simulink model "Validation_Kalman_Filters"  (R2019a)
settings: Solver=ode1  StartTime=0.0  StopTime=100  FixedStep=sampleTime  RelTol=1e-3
values from neighbouring files (symbols this model uses):
  bias = [0; 0; 1]    [Replay_Script.m]    (also in Validations_Script.m = [5; -3; 3]*pi/180)
  filter = d    [Replay_Script.m]    (also in Validations_Script.m = 3)
  Kalman_1 = Kalman_1_theta    [Replay_Script.m]    (also in Validations_Script.m = Setup_Kalman_1(Q, R, sampleTime))
  Kalman_2 = Kalman_2_theta    [Replay_Script.m]    (also in Validations_Script.m = Setup_Kalman_2(Q, R, sampleTime))
  Kalman_OP = Setup_Kalman_OP(Q, R)    [Replay_Script.m]    (also in Validations_Script.m)
  sampleTime = 0.05    [Replay_Script.m]    (also in Validations_Script.m)
undefined symbols (not defined in the file or in its folder): DiscIntNeverNeededParam
libraries: simulink x3
settings Model: Creator=Gaming  LastModifiedBy=Gaming

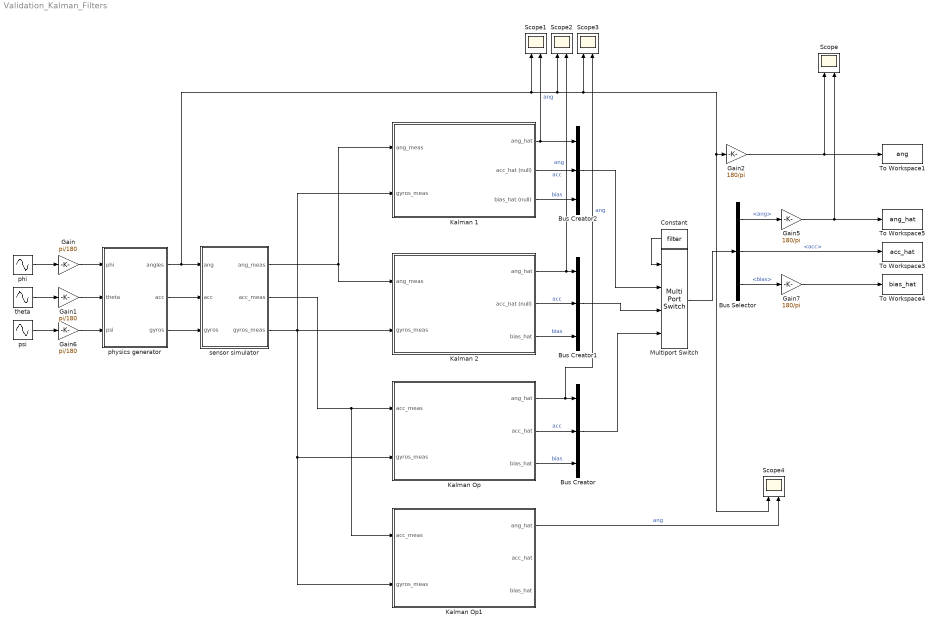
== system Validation_Kalman_Filters ==
  Bus Creator : BusCreator  Inputs=3
  Bus Creator1 : BusCreator  Inputs=3
  Bus Creator2 : BusCreator  Inputs=3
  Bus Selector : BusSelector  OutputSignals=ang,acc,bias
  Constant : Constant  Value=filter
  Gain : Gain  Gain=pi/180
  Gain1 : Gain  Gain=pi/180
  Gain2 : Gain  Gain=180/pi
  Gain5 : Gain  Gain=180/pi
  Gain6 : Gain  Gain=pi/180
  Gain7 : Gain  Gain=180/pi
  Kalman 1 : Subsystem
  Kalman 2 : Subsystem
  Kalman Op : Subsystem
  Kalman Op1 : Subsystem
  Multiport Switch : MultiPortSwitch  AllowDiffInputSizes=on
  Scope{,1..4} (5 alike) : Scope  NumInputPorts=2
  To Workspace1 : ToWorkspace  VariableName=ang  SaveFormat=Structure With Time  SampleTime=-1
  To Workspace3 : ToWorkspace  VariableName=acc_hat  SaveFormat=Structure With Time  SampleTime=-1
  To Workspace4 : ToWorkspace  VariableName=bias_hat  SaveFormat=Structure With Time  SampleTime=-1
  To Workspace5 : ToWorkspace  VariableName=ang_hat  SaveFormat=Structure With Time  SampleTime=-1
  phi : Sin  Amplitude=5  Bias=6  Frequency=2*pi/10  SampleTime=0
  physics generator : Subsystem
  psi : Sin  Amplitude=0  Bias=10  Frequency=2*pi/5  Phase=pi  SampleTime=0
  sensor simulator : Subsystem
  theta : Sin  Amplitude=10  Frequency=2*pi/5  Phase=pi  SampleTime=0
  wires:
  phi/1 -> Gain/1
  theta/1 -> Gain1/1
  Kalman Op/3(bias_hat) -> Bus Creator/3  "bias"
  Kalman Op/1(ang_hat) -> Scope3/2, Bus Creator/1  "ang"
  psi/1 -> Gain6/1
  Gain/1 -> physics generator/1(phi)
  Gain1/1 -> physics generator/2(theta)
  Gain6/1 -> physics generator/3(psi)
  physics generator/1(angles) -> sensor simulator/1(ang), Scope4/1, Gain2/1, Scope3/1, Scope2/1, Scope1/1
  physics generator/2(acc) -> sensor simulator/2(acc)
  physics generator/3(gyros) -> sensor simulator/3(gyros)
  Multiport Switch/1 -> Bus Selector/1
  Gain5/1 -> Scope/2, To Workspace5/1
  Gain7/1 -> To Workspace4/1
  Bus Selector/2 -> To Workspace3/1  "<acc>"
  Kalman Op/2(acc_hat) -> Bus Creator/2  "acc"
  Constant/1 -> Multiport Switch/1
  sensor simulator/2(acc_meas) -> Kalman Op1/1(acc_meas), Kalman Op/1(acc_meas)
  sensor simulator/3(gyros_meas) -> Kalman 2/2(gyros_meas), Kalman 1/2(gyros_meas), Kalman Op/2(gyros_meas), Kalman Op1/2(gyros_meas)
  Bus Selector/1 -> Gain5/1  "<ang>"
  Bus Selector/3 -> Gain7/1  "<bias>"
  Gain2/1 -> To Workspace1/1, Scope/1
  Bus Creator/1 -> Multiport Switch/4
  sensor simulator/1(ang_meas) -> Kalman 2/1(ang_meas), Kalman 1/1(ang_meas)
  Bus Creator1/1 -> Multiport Switch/3
  Bus Creator2/1 -> Multiport Switch/2
  Kalman 1/1(ang_hat) -> Bus Creator2/1, Scope1/2  "ang"
  Kalman 2/1(ang_hat) -> Scope2/2, Bus Creator1/1  "ang"
  Kalman 1/2(acc_hat (null)) -> Bus Creator2/2  "acc"
  Kalman 1/3(bias_hat (null)) -> Bus Creator2/3  "bias"
  Kalman 2/2(acc_hat (null)) -> Bus Creator1/2  "acc"
  Kalman 2/3(bias_hat) -> Bus Creator1/3  "bias"
  Kalman Op1/1(ang_hat) -> Scope4/2  "ang"

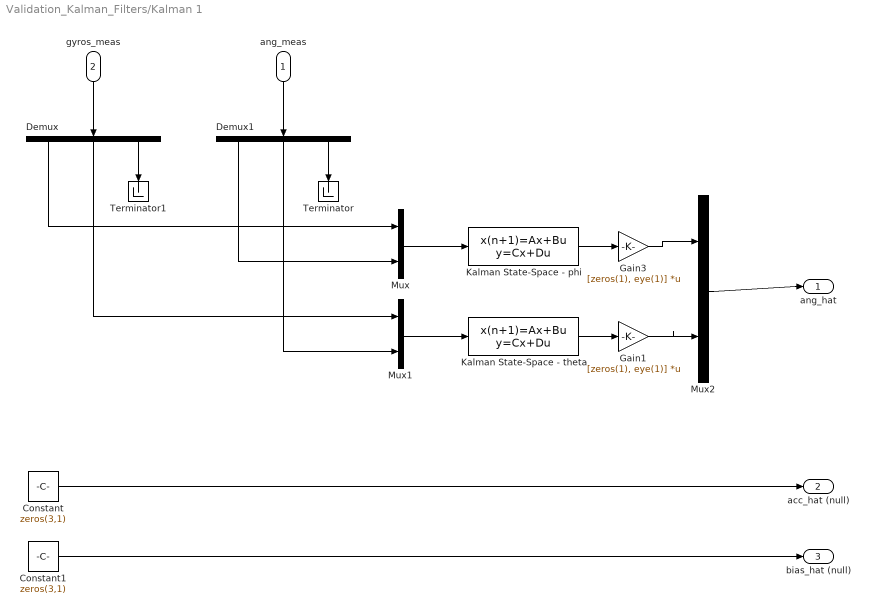
== system Validation_Kalman_Filters/Kalman 1 ==
  ang_meas : Inport
  gyros_meas : Inport  Port=2
  Constant : Constant  Value=zeros(3,1)
  Constant1 : Constant  Value=zeros(3,1)
  Demux : Demux  Outputs=3
  Demux1 : Demux  Outputs=3
  Gain1 : Gain  Gain=[zeros(1), eye(1)]  Multiplication=Matrix(K*u)
  Gain3 : Gain  Gain=[zeros(1), eye(1)]  Multiplication=Matrix(K*u)
  Kalman State-Space - phi : DiscreteStateSpace  A=Kalman_1.sys.A  B=Kalman_1.sys.B  C=Kalman_1.sys.C  D=Kalman_1.sys.D  SampleTime=-1
  Kalman State-Space - theta : DiscreteStateSpace  A=Kalman_1.sys.A  B=Kalman_1.sys.B  C=Kalman_1.sys.C  D=Kalman_1.sys.D  SampleTime=-1
  Mux : Mux  Inputs=2
  Mux1 : Mux  Inputs=2
  Mux2 : Mux  Inputs=2
  Terminator : Terminator
  Terminator1 : Terminator
  ang_hat : Outport  VectorParamsAs1DForOutWhenUnconnected=on
  acc_hat (null) : Outport  Port=2  VectorParamsAs1DForOutWhenUnconnected=on
  bias_hat (null) : Outport  Port=3  VectorParamsAs1DForOutWhenUnconnected=on
  wires:
  Kalman State-Space - phi/1 -> Gain3/1
  Mux/1 -> Kalman State-Space - phi/1
  Constant/1 -> acc_hat (null)/1
  Constant1/1 -> bias_hat (null)/1
  gyros_meas/1 -> Demux/1
  Kalman State-Space - theta/1 -> Gain1/1
  Mux1/1 -> Kalman State-Space - theta/1
  Mux2/1 -> ang_hat/1
  Gain3/1 -> Mux2/1
  Gain1/1 -> Mux2/2
  ang_meas/1 -> Demux1/1
  Demux1/3 -> Terminator/1
  Demux1/2 -> Mux1/2
  Demux1/1 -> Mux/2
  Demux/3 -> Terminator1/1
  Demux/1 -> Mux/1
  Demux/2 -> Mux1/1

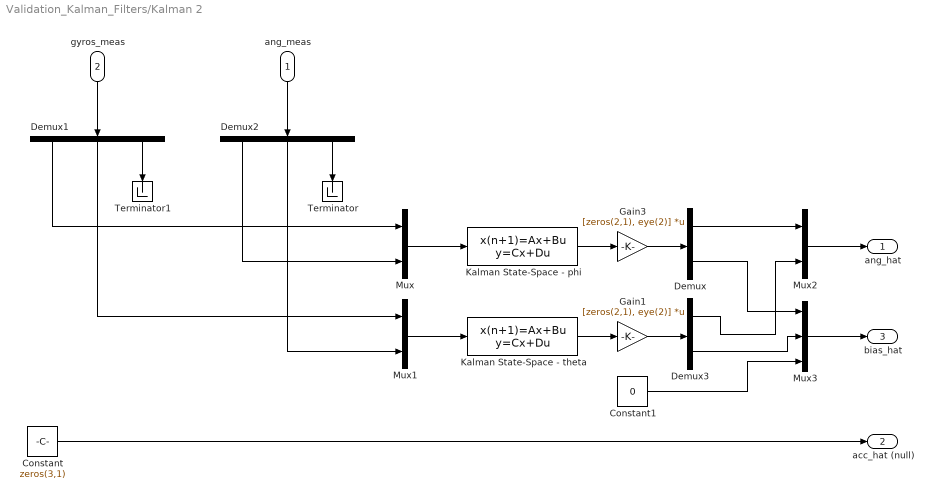
== system Validation_Kalman_Filters/Kalman 2 ==
  ang_meas : Inport
  gyros_meas : Inport  Port=2
  Constant : Constant  Value=zeros(3,1)
  Constant1 : Constant  Value=0
  Demux : Demux  Outputs=2
  Demux1 : Demux  Outputs=3
  Demux2 : Demux  Outputs=3
  Demux3 : Demux  Outputs=2
  Gain1 : Gain  Gain=[zeros(2,1), eye(2)]  Multiplication=Matrix(K*u)
  Gain3 : Gain  Gain=[zeros(2,1), eye(2)]  Multiplication=Matrix(K*u)
  Kalman State-Space - phi : DiscreteStateSpace  A=Kalman_2.sys.A  B=Kalman_2.sys.B  C=Kalman_2.sys.C  D=Kalman_2.sys.D  SampleTime=-1
  Kalman State-Space - theta : DiscreteStateSpace  A=Kalman_2.sys.A  B=Kalman_2.sys.B  C=Kalman_2.sys.C  D=Kalman_2.sys.D  SampleTime=-1
  Mux : Mux  Inputs=2
  Mux1 : Mux  Inputs=2
  Mux2 : Mux  Inputs=2
  Mux3 : Mux  Inputs=3
  Terminator : Terminator
  Terminator1 : Terminator
  ang_hat : Outport  VectorParamsAs1DForOutWhenUnconnected=on
  acc_hat (null) : Outport  Port=2  VectorParamsAs1DForOutWhenUnconnected=on
  bias_hat : Outport  Port=3  VectorParamsAs1DForOutWhenUnconnected=on
  wires:
  Kalman State-Space - phi/1 -> Gain3/1
  Gain3/1 -> Demux/1
  Constant/1 -> acc_hat (null)/1
  Demux2/2 -> Mux1/2
  Demux1/3 -> Terminator1/1
  ang_meas/1 -> Demux2/1
  Mux1/1 -> Kalman State-Space - theta/1
  Demux2/3 -> Terminator/1
  Mux/1 -> Kalman State-Space - phi/1
  gyros_meas/1 -> Demux1/1
  Demux2/1 -> Mux/2
  Kalman State-Space - theta/1 -> Gain1/1
  Gain1/1 -> Demux3/1
  Mux3/1 -> bias_hat/1
  Mux2/1 -> ang_hat/1
  Demux/1 -> Mux2/1
  Demux3/2 -> Mux3/2
  Demux1/2 -> Mux1/1
  Demux1/1 -> Mux/1
  Demux/2 -> Mux3/1
  Demux3/1 -> Mux2/2
  Constant1/1 -> Mux3/3

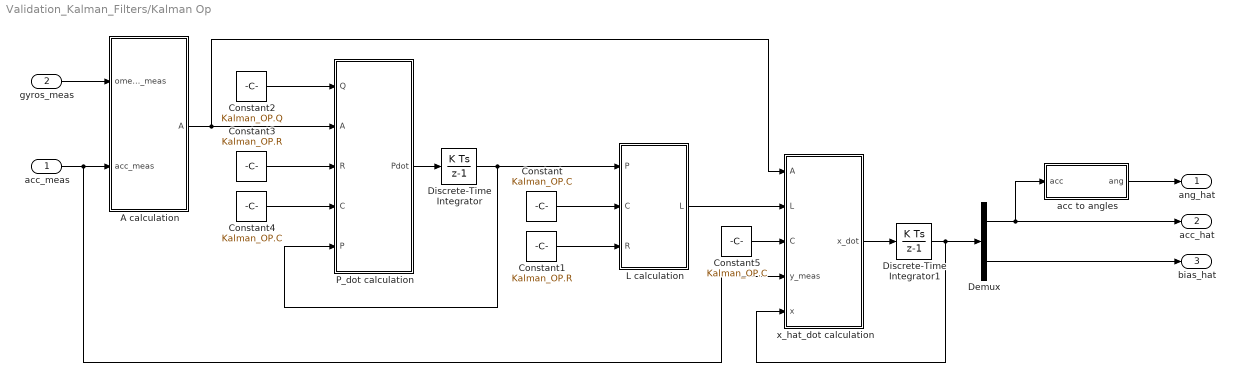
== system Validation_Kalman_Filters/Kalman Op ==
  acc_meas : Inport
  gyros_meas : Inport  Port=2
  A calculation : MATLAB Function  TreatAsAtomicUnit=on
  Constant : Constant  Value=Kalman_OP.C
  Constant1 : Constant  Value=Kalman_OP.R
  Constant2 : Constant  Value=Kalman_OP.Q
  Constant3 : Constant  Value=Kalman_OP.R
  Constant4 : Constant  Value=Kalman_OP.C
  Constant5 : Constant  Value=Kalman_OP.C
  Demux : Demux  Outputs=2
  Discrete-Time Integrator : DiscreteIntegrator  InitialCondition=Kalman_OP.Q*10  SampleTime=-1  ICPrevOutput=DiscIntNeverNeededParam  ICPrevScaledInput=DiscIntNeverNeededParam
  Discrete-Time Integrator1 : DiscreteIntegrator  InitialCondition=zeros(6,1)  SampleTime=-1  ICPrevOutput=DiscIntNeverNeededParam  ICPrevScaledInput=DiscIntNeverNeededParam
  L calculation : MATLAB Function  TreatAsAtomicUnit=on
  P_dot calculation : MATLAB Function  TreatAsAtomicUnit=on
  acc to angles : MATLAB Function  TreatAsAtomicUnit=on
  x_hat_dot calculation : MATLAB Function  TreatAsAtomicUnit=on
  ang_hat : Outport
  acc_hat : Outport  Port=2
  bias_hat : Outport  Port=3
  wires:
  acc to angles/1(ang) -> ang_hat/1
  x_hat_dot calculation/1(x_dot) -> Discrete-Time Integrator1/1
  Discrete-Time Integrator1/1 -> Demux/1, x_hat_dot calculation/5(x)
  L calculation/1(L) -> x_hat_dot calculation/2(L)
  P_dot calculation/1(Pdot) -> Discrete-Time Integrator/1
  Discrete-Time Integrator/1 -> P_dot calculation/5(P), L calculation/1(P)
  Constant/1 -> L calculation/2(C)
  Constant1/1 -> L calculation/3(R)
  Constant3/1 -> P_dot calculation/3(R)
  Constant2/1 -> P_dot calculation/1(Q)
  Demux/1 -> acc to angles/1(acc), acc_hat/1
  Demux/2 -> bias_hat/1
  acc_meas/1 -> x_hat_dot calculation/4(y_meas), A calculation/2(acc_meas)
  gyros_meas/1 -> A calculation/1(omega_meas)
  A calculation/1(A) -> x_hat_dot calculation/1(A), P_dot calculation/2(A)
  Constant4/1 -> P_dot calculation/4(C)
  Constant5/1 -> x_hat_dot calculation/3(C)

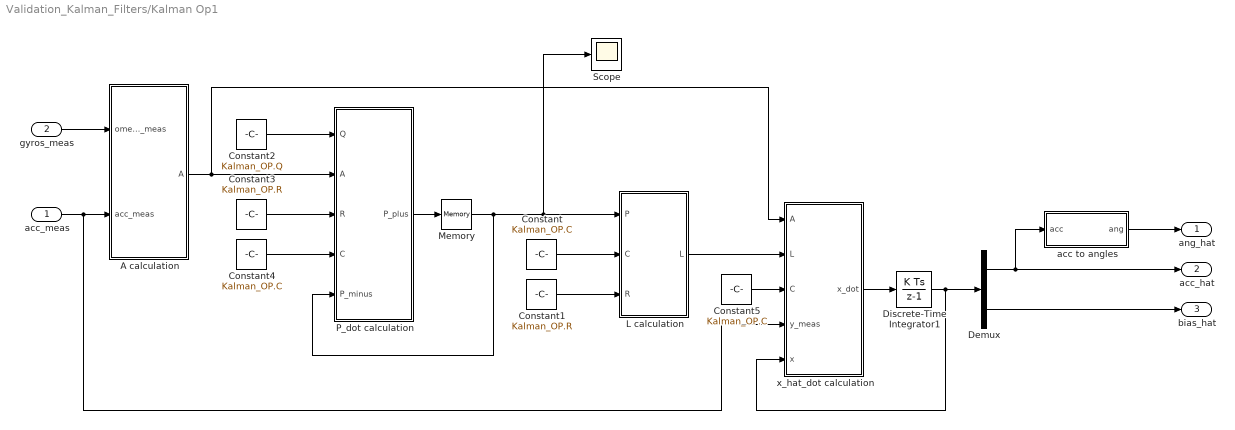
== system Validation_Kalman_Filters/Kalman Op1 ==
  acc_meas : Inport
  gyros_meas : Inport  Port=2
  A calculation : MATLAB Function  TreatAsAtomicUnit=on
  Constant : Constant  Value=Kalman_OP.C
  Constant1 : Constant  Value=Kalman_OP.R
  Constant2 : Constant  Value=Kalman_OP.Q
  Constant3 : Constant  Value=Kalman_OP.R
  Constant4 : Constant  Value=Kalman_OP.C
  Constant5 : Constant  Value=Kalman_OP.C
  Demux : Demux  Outputs=2
  Discrete-Time Integrator1 : DiscreteIntegrator  InitialCondition=zeros(6,1)  SampleTime=-1  ICPrevOutput=DiscIntNeverNeededParam  ICPrevScaledInput=DiscIntNeverNeededParam
  L calculation : MATLAB Function  TreatAsAtomicUnit=on
  Memory : Memory  InitialCondition=Kalman_OP.Q*10  InheritSampleTime=on
  P_dot calculation : MATLAB Function  TreatAsAtomicUnit=on
  Scope : Scope
  acc to angles : MATLAB Function  TreatAsAtomicUnit=on
  x_hat_dot calculation : MATLAB Function  TreatAsAtomicUnit=on
  ang_hat : Outport
  acc_hat : Outport  Port=2
  bias_hat : Outport  Port=3
  wires:
  acc to angles/1(ang) -> ang_hat/1
  x_hat_dot calculation/1(x_dot) -> Discrete-Time Integrator1/1
  Discrete-Time Integrator1/1 -> Demux/1, x_hat_dot calculation/5(x)
  L calculation/1(L) -> x_hat_dot calculation/2(L)
  P_dot calculation/1(P_plus) -> Memory/1
  Constant/1 -> L calculation/2(C)
  Constant1/1 -> L calculation/3(R)
  Constant3/1 -> P_dot calculation/3(R)
  Constant2/1 -> P_dot calculation/1(Q)
  Demux/1 -> acc to angles/1(acc), acc_hat/1
  Demux/2 -> bias_hat/1
  acc_meas/1 -> x_hat_dot calculation/4(y_meas), A calculation/2(acc_meas)
  gyros_meas/1 -> A calculation/1(omega_meas)
  A calculation/1(A) -> x_hat_dot calculation/1(A), P_dot calculation/2(A)
  Constant4/1 -> P_dot calculation/4(C)
  Constant5/1 -> x_hat_dot calculation/3(C)
  Memory/1 -> P_dot calculation/5(P_minus), Scope/1, L calculation/1(P)

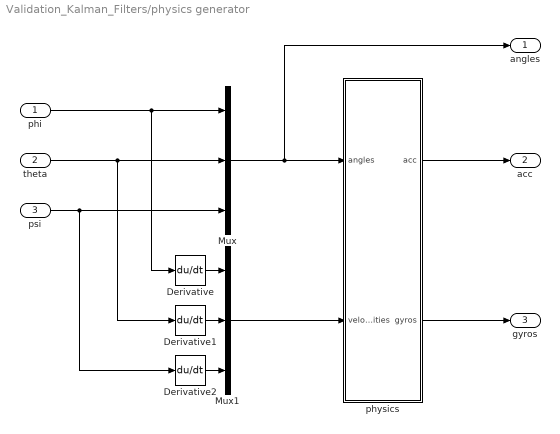
== system Validation_Kalman_Filters/physics generator ==
  phi : Inport
  theta : Inport  Port=2
  psi : Inport  Port=3
  Derivative : Derivative
  Derivative1 : Derivative
  Derivative2 : Derivative
  Mux : Mux  Inputs=3
  Mux1 : Mux  Inputs=3
  physics : MATLAB Function  TreatAsAtomicUnit=on
  angles : Outport
  acc : Outport  Port=2
  gyros : Outport  Port=3
  wires:
  phi/1 -> Derivative/1, Mux/1
  Derivative2/1 -> Mux1/3
  psi/1 -> Derivative2/1, Mux/3
  physics/1(acc) -> acc/1
  theta/1 -> Derivative1/1, Mux/2
  Mux/1 -> angles/1, physics/1(angles)
  Derivative1/1 -> Mux1/2
  Derivative/1 -> Mux1/1
  Mux1/1 -> physics/2(velocities)
  physics/2(gyros) -> gyros/1

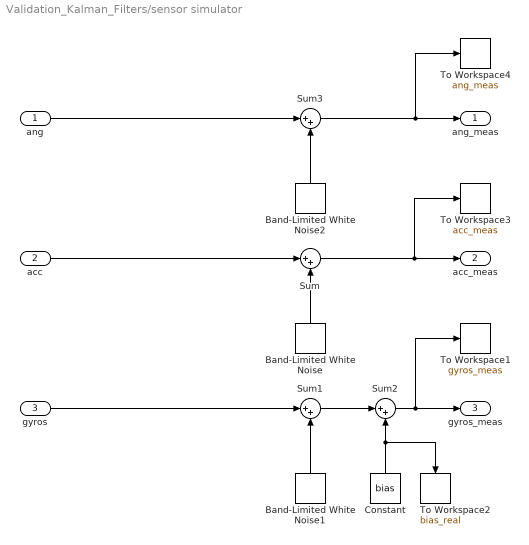
== system Validation_Kalman_Filters/sensor simulator ==
  ang : Inport
  acc : Inport  Port=2
  gyros : Inport  Port=3
  Band-Limited White Noise : simulink/Sources/Band-Limited White Noise  Cov=[0.05^2*sampleTime]  Ts=sampleTime  seed=[23331]
  Band-Limited White Noise1 : simulink/Sources/Band-Limited White Noise  Cov=[(0.05*pi/180)^2*sampleTime]  Ts=sampleTime  seed=[23341]
  Band-Limited White Noise2 : simulink/Sources/Band-Limited White Noise  Cov=[0.05^2*sampleTime]  Ts=sampleTime  seed=[23331]
  Constant : Constant  Value=bias  VectorParams1D=off
  Sum{,1..3} (4 alike) : Sum  Inputs=|++
  To Workspace1 : ToWorkspace  VariableName=gyros_meas  SaveFormat=Structure With Time  SampleTime=-1
  To Workspace2 : ToWorkspace  VariableName=bias_real  SaveFormat=Structure With Time  SampleTime=-1
  To Workspace3 : ToWorkspace  VariableName=acc_meas  SaveFormat=Structure With Time  SampleTime=-1
  To Workspace4 : ToWorkspace  VariableName=ang_meas  SaveFormat=Structure With Time  SampleTime=-1
  ang_meas : Outport
  acc_meas : Outport  Port=2
  gyros_meas : Outport  Port=3
  wires:
  acc/1 -> Sum/1
  Constant/1 -> To Workspace2/1, Sum2/2
  Sum2/1 -> gyros_meas/1, To Workspace1/1
  Sum1/1 -> Sum2/1
  Sum/1 -> To Workspace3/1, acc_meas/1
  gyros/1 -> Sum1/1
  Sum3/1 -> To Workspace4/1, ang_meas/1
  ang/1 -> Sum3/1
  Band-Limited White Noise2/1 -> Sum3/2
  Band-Limited White Noise/1 -> Sum/2
  Band-Limited White Noise1/1 -> Sum1/2

== matlab function Validation_Kalman_Filters/Kalman Op/P_dot calculation ==
  data: Q input; A input; Pdot output; R input; C input; P input
function Pdot = fcn(Q, A, R, C, P)

Pdot = A*P + P*transpose(A) + Q - P*transpose(C)*inv(R)*C*P;

== matlab function Validation_Kalman_Filters/physics generator/physics ==
  data: angles input; acc output; velocities input; gyros output
function [acc,gyros] = fcn(angles, velocities)

% angles - phi, theta

acc = -10*[-sin(angles(2)); cos(angles(2))*sin(angles(1));cos(angles(2))*cos(angles(1))];

A = [1, sin(velocities(1))*tan(velocities(2))   , cos(velocities(1))*tan(velocities(2)) ;...
     0, cos(velocities(1))                      , -sin(velocities(1))                   ;...
     0, sin(velocities(1))/cos(velocities(2))   , cos(velocities(1))/cos(velocities(2))];


gyros = A\[velocities];

== matlab function Validation_Kalman_Filters/Kalman Op/acc to angles ==
  data: acc input; ang output
function ang = fcn(acc)

phi = -atan2(acc(2),-acc(3));

theta = atan2(acc(1),sqrt(acc(2)^2+acc(3)^2));

ang = [phi; theta];

== matlab function Validation_Kalman_Filters/Kalman Op/L calculation ==
  data: P input; L output; C input; R input
function L = fcn(P, C, R)

L = P*transpose(C)*inv(R);

== matlab function Validation_Kalman_Filters/Kalman Op/x_hat_dot calculation ==
  data: A input; x_dot output; L input; C input; y_meas input; x input
function x_dot = fcn(A,L,C,y_meas,x)

x_dot = A*x + L*(y_meas - C*x);

== matlab function Validation_Kalman_Filters/Kalman Op/A calculation ==
  data: omega_meas input; A output; acc_meas input
function A = fcn(omega_meas, acc_meas)

w = omega_meas;
a = acc_meas;

s_1 = [ 0   , -w(3) ,  w(2) ;...
        w(3),  0    , -w(1) ;...
       -w(2),  w(1) ,  0    ];
   
s_2 = [ 0   , -a(3) ,  a(2) ;...
        a(3),  0    , -a(1) ;...
       -a(2),  a(1) ,  0    ];
   
A = [-s_1, -s_2 ;...
     zeros(3,6) ];

== matlab function Validation_Kalman_Filters/Kalman Op1/A calculation ==
  data: omega_meas input; A output; acc_meas input
function A = fcn(omega_meas, acc_meas)

w = omega_meas;
a = acc_meas;

s_1 = [ 0   , -w(3) ,  w(2) ;...
        w(3),  0    , -w(1) ;...
       -w(2),  w(1) ,  0    ];
   
s_2 = [ 0   , -a(3) ,  a(2) ;...
        a(3),  0    , -a(1) ;...
       -a(2),  a(1) ,  0    ];
   
A = [-s_1, -s_2 ;...
     zeros(3,6) ];

== matlab function Validation_Kalman_Filters/Kalman Op1/L calculation ==
  data: P input; L output; C input; R input
function L = fcn(P, C, R)

L = P*transpose(C)*inv(R);

== matlab function Validation_Kalman_Filters/Kalman Op1/P_dot calculation ==
  data: Q input; A input; P_plus output; R input; C input; P_minus input
function P_plus = fcn(Q, A, R, C, P_minus)

sampleTime = 0.05;

A_d = eye(6) + A*sampleTime + A^2*sampleTime^2/2;

P_plus = A_d*P_minus*transpose(A_d) + Q*sampleTime^2 -...
         P_minus*transpose(C)*inv(R)*C*P_minus*sampleTime;

== matlab function Validation_Kalman_Filters/Kalman Op1/acc to angles ==
  data: acc input; ang output
function ang = fcn(acc)

phi = -atan2(acc(2),-acc(3));

theta = atan2(acc(1),sqrt(acc(2)^2+acc(3)^2));

ang = [phi; theta];

== matlab function Validation_Kalman_Filters/Kalman Op1/x_hat_dot calculation ==
  data: A input; x_dot output; L input; C input; y_meas input; x input
function x_dot = fcn(A,L,C,y_meas,x)

x_dot = A*x + L*(y_meas - C*x);
